simulink model "fdii_continuo"  (R2026a)
settings: Solver=VariableStepAuto  StopTime=2  MaxStep=0.001

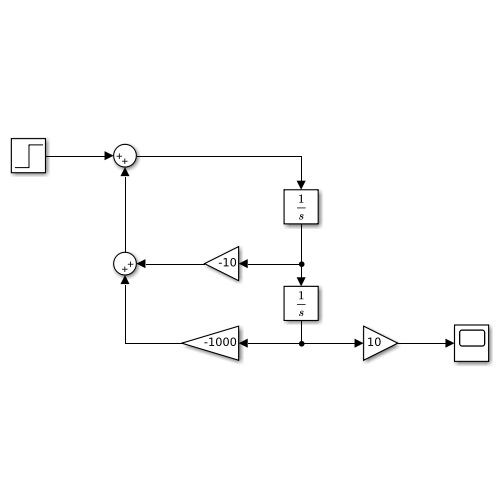
[thumbnail: Simulink's stored preview of the top-level diagram]
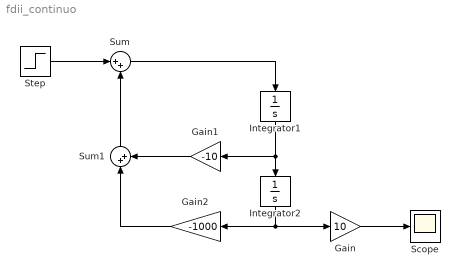
== system fdii_continuo ==
  Gain : Gain  Gain=10
  Gain1 : Gain  Gain=-10
  Gain2 : Gain  Gain=-1000
  Integrator1 : Integrator
  Integrator2 : Integrator
  Scope : Scope
      settings: ActiveDisplayYMinimum=-0.020058487824574926  ActiveDisplayYMaximum=0.18052639042117435
  Step : Step  Time=0  FinalValue=10  SampleTime=0
  Sum : Sum  Inputs=|++
  Sum1 : Sum  Inputs=|++
  wires:
  Step/1 -> Sum/1
  Sum/1 -> Integrator1/1
  Sum1/1 -> Sum/2
  Integrator1/1 -> Gain1/1, Integrator2/1
  Gain2/1 -> Sum1/1
  Gain1/1 -> Sum1/2
  Integrator2/1 -> Gain2/1, Gain/1
  Gain/1 -> Scope/1
